simulink model "DeadbeatSISO"  (R2016b)
settings: Solver=VariableStepAuto  StartTime=0.0  StopTime=10.0  RelTol=1e-3
values from neighbouring files (symbols this model uses):
  s = tf('s')    [DeadbeatDesignerSS.m]
undefined symbols (not defined in the file or in its folder): z
libraries: cstblocks x2
settings Model: Creator=capn  LastModifiedBy=capn

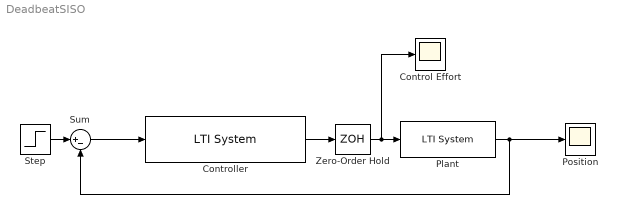
== system DeadbeatSISO ==
  Control Effort : Scope
  Controller : cstblocks/LTI System  sys=(1.5820*z-0.5820)/(z+0.4180)  IC=[]
  Plant : cstblocks/LTI System  sys=1/s/(s+1)  IC=[]
  Position : Scope
  Step : Step  Time=0  SampleTime=0
  Sum : Sum  Inputs=|+-
  Zero-Order Hold : ZeroOrderHold  SampleTime=-1
  wires:
  Controller/1 -> Zero-Order Hold/1
  Zero-Order Hold/1 -> Control Effort/1, Plant/1
  Step/1 -> Sum/1
  Plant/1 -> Position/1, Sum/2
  Sum/1 -> Controller/1
